simulink model "therm_model2"  (Simulink 7.5)
settings: Solver=ode45  StartTime=0.0  StopTime=48  RelTol=1e-3  AbsTol=1e-6
libraries: simulink x1
settings Model: Creator=gregfiore  LastModifiedBy=gregfiore
settings DebuggingCC: SolverPrmCheckMsg=none

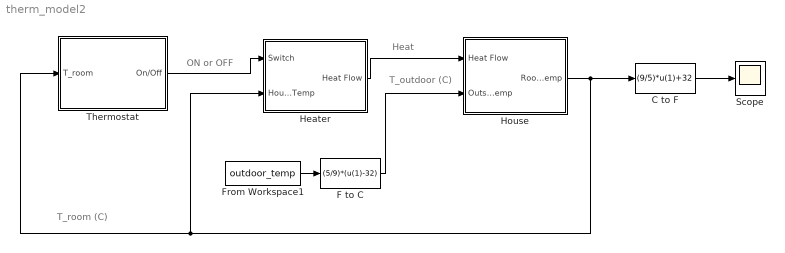
== system therm_model2 ==
  note: T_room (C)
  note: ON or OFF
  note: T_outdoor (C)
  note: Heat
  C to F : Fcn  Expr=(9/5)*u(1)+32
  F to C : Fcn  Expr=(5/9)*(u(1)-32)
  From Workspace1 : FromWorkspace  VariableName=outdoor_temp  SampleTime=0
  Heater : Subsystem
  House : Subsystem
  Scope : Scope
  Thermostat : Subsystem
      mask Display:
      | a = imread('nest_thermostat.jpg');
      | b = 256*ones(383,137,3);
      | 
      | e = [b, a, b];
      | 
      | f = 256*ones(40, size(e,2), 3);
      | 
      | img = [f;e;f];
      | 
      | image(img)
  wires:
  Thermostat/1(On/Off) -> Heater/1(Switch)
  Heater/1(Heat Flow) -> House/1(Heat Flow)
  House/1(Room Temp) -> C to F/1, Heater/2(House Temp), Thermostat/1(T_room)
  F to C/1 -> House/2(Outside Temp)
  C to F/1 -> Scope/1
  From Workspace1/1 -> F to C/1

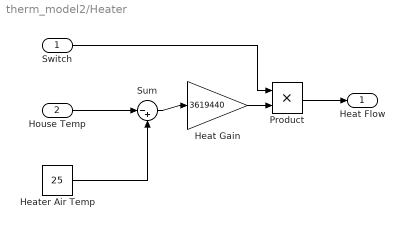
== system therm_model2/Heater ==
  Switch : Inport  OutDataType=fixdt(1, 16)  OutScaling=2^0
  House Temp : Inport  Port=2  OutDataType=fixdt(1, 16)  OutScaling=2^0
  Heat Gain : Gain  Gain=3619440  ParameterDataType=fixdt(1, 16)  ParameterScaling=2^0  OutDataType=fixdt(1, 16)  OutScaling=2^0
  Heater Air Temp : Constant  Value=25  OutDataType=fixdt(1, 16)  OutScaling=2^0
  Product : Product  OutDataType=fixdt(1, 16)  OutScaling=2^0  RndMeth=Zero
  Sum : Sum  Inputs=|-+  OutDataType=fixdt(1, 16)  OutScaling=2^0
  Heat Flow : Outport  OutDataType=fixdt(1, 16)  OutScaling=2^0
  wires:
  House Temp/1 -> Sum/1
  Heater Air Temp/1 -> Sum/2
  Sum/1 -> Heat Gain/1
  Heat Gain/1 -> Product/2
  Switch/1 -> Product/1
  Product/1 -> Heat Flow/1

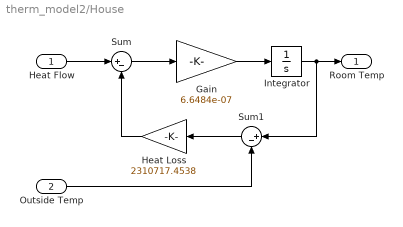
== system therm_model2/House ==
  Heat Flow : Inport  OutDataType=fixdt(1, 16)  OutScaling=2^0
  Outside Temp : Inport  Port=2  OutDataType=fixdt(1, 16)  OutScaling=2^0
  Gain : Gain  Gain=6.6484e-07  ParameterDataType=fixdt(1, 16)  ParameterScaling=2^0  OutDataType=fixdt(1, 16)  OutScaling=2^0  SampleTime=1/60
  Heat Loss : Gain  Gain=2310717.4538  ParameterDataType=fixdt(1, 16)  ParameterScaling=2^0  OutDataType=fixdt(1, 16)  OutScaling=2^0  SampleTime=1/60
  Integrator : Integrator  InitialCondition=21.1111
  Sum : Sum  Inputs=|+-  OutDataType=fixdt(1, 16)  OutScaling=2^0
  Sum1 : Sum  Inputs=|+-  OutDataType=fixdt(1, 16)  OutScaling=2^0
  Room Temp : Outport  OutDataType=fixdt(1, 16)  OutScaling=2^0
  wires:
  Sum/1 -> Gain/1
  Heat Flow/1 -> Sum/1
  Integrator/1 -> Room Temp/1, Sum1/1
  Gain/1 -> Integrator/1
  Outside Temp/1 -> Sum1/2
  Sum1/1 -> Heat Loss/1
  Heat Loss/1 -> Sum/2

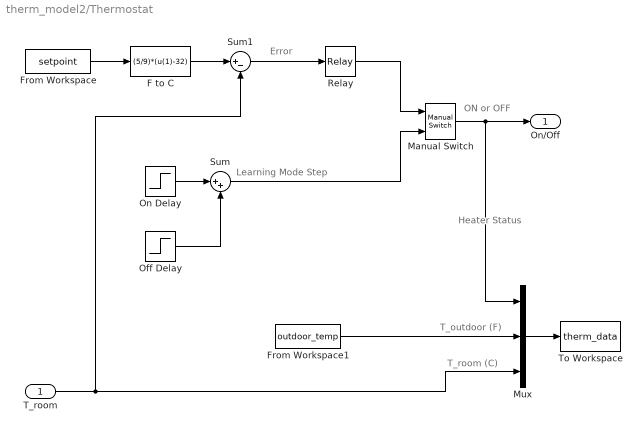
== system therm_model2/Thermostat ==
  note: ON or OFF
  note: T_outdoor (F)
  note: T_room (C)
  note: Learning Mode Step
  note: Heater Status
  note: Error
  T_room : Inport  OutDataType=fixdt(1, 16)  OutScaling=2^0
  F to C : Fcn  Expr=(5/9)*(u(1)-32)
  From Workspace : FromWorkspace  VariableName=setpoint  SampleTime=1
  From Workspace1 : FromWorkspace  VariableName=outdoor_temp  SampleTime=0
  Manual Switch : simulink/Signal Routing/Manual Switch  SystemSampleTime=-1  sw=0  action=0  varsize=off
  Mux : Mux  Inputs=3
  Off Delay : Step  After=-1  SampleTime=0
  On Delay : Step  Time=0.5  SampleTime=0
  Relay : Relay  OnSwitchValue=4*(5/9)  OffSwitchValue=-4*(5/9)  OutDataType=fixdt(1, 16)  OutScaling=2^0
  Sum : Sum  Inputs=|++  OutDataType=fixdt(1, 16)  OutScaling=2^0
  Sum1 : Sum  Inputs=|+-  OutDataType=fixdt(1, 16)  OutScaling=2^0
  To Workspace : ToWorkspace  VariableName=therm_data  SampleTime=-1  SaveFormat=Structure With Time
  On/Off : Outport  OutDataType=fixdt(1, 16)  OutScaling=2^0
  wires:
  On Delay/1 -> Sum/1
  Off Delay/1 -> Sum/2
  Mux/1 -> To Workspace/1
  From Workspace1/1 -> Mux/2
  T_room/1 -> Mux/3, Sum1/2
  From Workspace/1 -> F to C/1
  F to C/1 -> Sum1/1
  Sum1/1 -> Relay/1
  Relay/1 -> Manual Switch/1
  Manual Switch/1 -> On/Off/1, Mux/1
  Sum/1 -> Manual Switch/2
